simulink model "gm_final_heart_sym2_level4_hdl"  (R2021a)
settings: Solver=FixedStepDiscrete  StartTime=0.0  StopTime=8  RelTol=1e-3
libraries: hdlmdlgenlib x45
(part 2 of 3)

== system gm_final_heart_sym2_level4_hdl/DWT_Sym2_Level4/1st_Level_Decomp/LoD_Even ==
  In_LoD_e : Inport  OutDataTypeStr=fixdt(0, 16, 23)  PortDimensions=1  SampleTime=2.26757369614512e-05
  Add : Sum  AccumDataTypeStr=fixdt(1, 16, 22)  OutDataTypeStr=fixdt(1, 16, 23)  SampleTime=2.26757369614512e-05
  Delay : Delay  DelayLength=double(1)  InitialCondition=0  SampleTime=2.26757369614512e-05
  HwModeRegister{,1..3} (4 alike) : Delay  DelayLength=double(1)  InitialCondition=0  SampleTime=2.26757369614512e-05
  LoD_0 : Constant  Value=-0.1294097900390625  OutDataTypeStr=fixdt(1, 16, 17)  SampleTime=2.26757369614512e-05
  LoD_2 : Constant  Value=0.836517333984375  OutDataTypeStr=fixdt(0, 16, 16)  SampleTime=2.26757369614512e-05
  Multiply : Product  Inputs=**  OutDataTypeStr=fixdt(1, 16, 15)  SampleTime=2.26757369614512e-05
  Multiply1 : Product  Inputs=**  OutDataTypeStr=fixdt(0, 16, 23)  SampleTime=2.26757369614512e-05
  PipelineRegister : Delay  DelayLength=double(1)  InitialCondition=0  SampleTime=2.26757369614512e-05
  PipelineRegister1 : Delay  DelayLength=double(1)  InitialCondition=0  SampleTime=2.26757369614512e-05
  Rate Transition : hdlmdlgenlib/Buffer
      settings: SourceProductBaseCode=SL
  delayMatch : Delay  DelayLength=double(1)  InitialCondition=0  SampleTime=2.26757369614512e-05
  Out_LoD_e : Outport  OutDataTypeStr=fixdt(1,16,23)  SampleTime=2.26757369614512e-05  VectorParamsAs1DForOutWhenUnconnected=off
  wires:
  Add/1 -> Out_LoD_e/1
  Delay/1 -> Rate Transition/1
  LoD_0/1 -> HwModeRegister/1
  LoD_2/1 -> HwModeRegister2/1
  PipelineRegister/1 -> Add/1
  delayMatch/1 -> Add/2
  Rate Transition/1 -> HwModeRegister3/1
  In_LoD_e/1 -> Delay/1, HwModeRegister1/1
  PipelineRegister1/1 -> delayMatch/1
  Multiply/1 -> PipelineRegister/1
  HwModeRegister/1 -> Multiply/1
  HwModeRegister1/1 -> Multiply/2
  Multiply1/1 -> PipelineRegister1/1
  HwModeRegister2/1 -> Multiply1/1
  HwModeRegister3/1 -> Multiply1/2

== system gm_final_heart_sym2_level4_hdl/DWT_Sym2_Level4/1st_Level_Decomp/LoD_Odd ==
  In_LoD_o : Inport  OutDataTypeStr=fixdt(0, 16, 23)  PortDimensions=1  SampleTime=2.26757369614512e-05
  Add : Sum  AccumDataTypeStr=fixdt(0, 16, 24)  OutDataTypeStr=fixdt(0, 16, 24)  SampleTime=2.26757369614512e-05
  Delay : Delay  DelayLength=double(1)  InitialCondition=0  SampleTime=2.26757369614512e-05
  HwModeRegister{,1..3} (4 alike) : Delay  DelayLength=double(1)  InitialCondition=0  SampleTime=2.26757369614512e-05
  LoD_1 : Constant  Value=0.22414398193359375  OutDataTypeStr=fixdt(0, 16, 18)  SampleTime=2.26757369614512e-05
  LoD_3 : Constant  Value=0.48296356201171875  OutDataTypeStr=fixdt(0, 16, 17)  SampleTime=2.26757369614512e-05
  Multiply : Product  Inputs=**  OutDataTypeStr=fixdt(0, 16, 25)  SampleTime=2.26757369614512e-05
  Multiply1 : Product  Inputs=**  OutDataTypeStr=fixdt(0, 16, 24)  SampleTime=2.26757369614512e-05
  PipelineRegister : Delay  DelayLength=double(1)  InitialCondition=0  SampleTime=2.26757369614512e-05
  PipelineRegister1 : Delay  DelayLength=double(1)  InitialCondition=0  SampleTime=2.26757369614512e-05
  Rate Transition : hdlmdlgenlib/Buffer
      settings: SourceProductBaseCode=SL
  delayMatch : Delay  DelayLength=double(1)  InitialCondition=0  SampleTime=2.26757369614512e-05
  Out_LoD_o : Outport  OutDataTypeStr=fixdt(0,16,24)  SampleTime=2.26757369614512e-05  VectorParamsAs1DForOutWhenUnconnected=off
  wires:
  Add/1 -> Out_LoD_o/1
  Delay/1 -> Rate Transition/1
  LoD_1/1 -> HwModeRegister/1
  LoD_3/1 -> HwModeRegister2/1
  PipelineRegister/1 -> Add/1
  delayMatch/1 -> Add/2
  Rate Transition/1 -> HwModeRegister3/1
  In_LoD_o/1 -> Delay/1, HwModeRegister1/1
  PipelineRegister1/1 -> delayMatch/1
  Multiply/1 -> PipelineRegister/1
  HwModeRegister/1 -> Multiply/1
  HwModeRegister1/1 -> Multiply/2
  Multiply1/1 -> PipelineRegister1/1
  HwModeRegister2/1 -> Multiply1/1
  HwModeRegister3/1 -> Multiply1/2

== system gm_final_heart_sym2_level4_hdl/DWT_Sym2_Level4/1st_Level_Decomp1/HiD_Even ==
  In_HiD_e : Inport  OutDataTypeStr=fixdt(1, 16, 22)  PortDimensions=1  SampleTime=2.26757369614512e-05
  Add : Sum  AccumDataTypeStr=fixdt(1, 16, 15)  OutDataTypeStr=fixdt(1, 16, 15)  SampleTime=2.26757369614512e-05
  Delay : Delay  DelayLength=double(1)  InitialCondition=0  SampleTime=2.26757369614512e-05
  HiD_0 : Constant  Value=-0.4829559326171875  OutDataTypeStr=fixdt(1, 16, 16)  SampleTime=2.26757369614512e-05
  HiD_2 : Constant  Value=-0.22414398193359375  OutDataTypeStr=fixdt(1, 16, 17)  SampleTime=2.26757369614512e-05
  HwModeRegister{,1..3} (4 alike) : Delay  DelayLength=double(1)  InitialCondition=0  SampleTime=2.26757369614512e-05
  Multiply : Product  Inputs=**  OutDataTypeStr=fixdt(1, 16, 15)  SampleTime=2.26757369614512e-05
  Multiply1 : Product  Inputs=**  OutDataTypeStr=fixdt(1, 16, 15)  SampleTime=2.26757369614512e-05
  PipelineRegister : Delay  DelayLength=double(1)  InitialCondition=0  SampleTime=2.26757369614512e-05
  PipelineRegister1 : Delay  DelayLength=double(1)  InitialCondition=0  SampleTime=2.26757369614512e-05
  Rate Transition : hdlmdlgenlib/Buffer
      settings: SourceProductBaseCode=SL
  delayMatch : Delay  DelayLength=double(1)  InitialCondition=0  SampleTime=2.26757369614512e-05
  Out_HiD_e : Outport  OutDataTypeStr=fixdt(1,16,15)  SampleTime=2.26757369614512e-05  VectorParamsAs1DForOutWhenUnconnected=off
  wires:
  Add/1 -> Out_HiD_e/1
  Delay/1 -> Rate Transition/1
  HiD_0/1 -> HwModeRegister/1
  HiD_2/1 -> HwModeRegister2/1
  PipelineRegister/1 -> Add/1
  delayMatch/1 -> Add/2
  Rate Transition/1 -> HwModeRegister3/1
  In_HiD_e/1 -> Delay/1, HwModeRegister1/1
  PipelineRegister1/1 -> delayMatch/1
  Multiply/1 -> PipelineRegister/1
  HwModeRegister/1 -> Multiply/1
  HwModeRegister1/1 -> Multiply/2
  Multiply1/1 -> PipelineRegister1/1
  HwModeRegister2/1 -> Multiply1/1
  HwModeRegister3/1 -> Multiply1/2

== system gm_final_heart_sym2_level4_hdl/DWT_Sym2_Level4/1st_Level_Decomp1/HiD_Odd ==
  In_HiD_o : Inport  OutDataTypeStr=fixdt(1, 16, 22)  PortDimensions=1  SampleTime=2.26757369614512e-05
  Add : Sum  AccumDataTypeStr=fixdt(1, 16, 23)  OutDataTypeStr=fixdt(1, 16, 23)  SampleTime=2.26757369614512e-05
  Delay : Delay  DelayLength=double(1)  InitialCondition=0  SampleTime=2.26757369614512e-05
  HiD_1 : Constant  Value=0.836517333984375  OutDataTypeStr=fixdt(0, 16, 16)  SampleTime=2.26757369614512e-05
  HiD_3 : Constant  Value=-0.1294097900390625  OutDataTypeStr=fixdt(1, 16, 17)  SampleTime=2.26757369614512e-05
  HwModeRegister{,1..3} (4 alike) : Delay  DelayLength=double(1)  InitialCondition=0  SampleTime=2.26757369614512e-05
  Multiply : Product  Inputs=**  OutDataTypeStr=fixdt(0, 16, 24)  SampleTime=2.26757369614512e-05
  Multiply1 : Product  Inputs=**  OutDataTypeStr=fixdt(1, 16, 15)  SampleTime=2.26757369614512e-05
  PipelineRegister : Delay  DelayLength=double(1)  InitialCondition=0  SampleTime=2.26757369614512e-05
  PipelineRegister1 : Delay  DelayLength=double(1)  InitialCondition=0  SampleTime=2.26757369614512e-05
  Rate Transition : hdlmdlgenlib/Buffer
      settings: SourceProductBaseCode=SL
  delayMatch : Delay  DelayLength=double(1)  InitialCondition=0  SampleTime=2.26757369614512e-05
  Out_HiD_o : Outport  OutDataTypeStr=fixdt(1,16,23)  SampleTime=2.26757369614512e-05  VectorParamsAs1DForOutWhenUnconnected=off
  wires:
  Add/1 -> Out_HiD_o/1
  Delay/1 -> Rate Transition/1
  HiD_1/1 -> HwModeRegister/1
  HiD_3/1 -> HwModeRegister2/1
  PipelineRegister/1 -> Add/1
  delayMatch/1 -> Add/2
  Rate Transition/1 -> HwModeRegister3/1
  In_HiD_o/1 -> Delay/1, HwModeRegister1/1
  PipelineRegister1/1 -> delayMatch/1
  Multiply/1 -> PipelineRegister/1
  HwModeRegister/1 -> Multiply/1
  HwModeRegister1/1 -> Multiply/2
  Multiply1/1 -> PipelineRegister1/1
  HwModeRegister2/1 -> Multiply1/1
  HwModeRegister3/1 -> Multiply1/2

== system gm_final_heart_sym2_level4_hdl/DWT_Sym2_Level4/1st_Level_Decomp1/LoD_Even ==
  In_LoD_e : Inport  OutDataTypeStr=fixdt(1, 16, 22)  PortDimensions=1  SampleTime=2.26757369614512e-05
  Add : Sum  AccumDataTypeStr=fixdt(1, 16, 23)  OutDataTypeStr=fixdt(1, 16, 23)  SampleTime=2.26757369614512e-05
  Delay : Delay  DelayLength=double(1)  InitialCondition=0  SampleTime=2.26757369614512e-05
  HwModeRegister{,1..3} (4 alike) : Delay  DelayLength=double(1)  InitialCondition=0  SampleTime=2.26757369614512e-05
  LoD_0 : Constant  Value=-0.1294097900390625  OutDataTypeStr=fixdt(1, 16, 17)  SampleTime=2.26757369614512e-05
  LoD_2 : Constant  Value=0.836517333984375  OutDataTypeStr=fixdt(0, 16, 16)  SampleTime=2.26757369614512e-05
  Multiply : Product  Inputs=**  OutDataTypeStr=fixdt(1, 16, 15)  SampleTime=2.26757369614512e-05
  Multiply1 : Product  Inputs=**  OutDataTypeStr=fixdt(0, 16, 24)  SampleTime=2.26757369614512e-05
  PipelineRegister : Delay  DelayLength=double(1)  InitialCondition=0  SampleTime=2.26757369614512e-05
  PipelineRegister1 : Delay  DelayLength=double(1)  InitialCondition=0  SampleTime=2.26757369614512e-05
  Rate Transition : hdlmdlgenlib/Buffer
      settings: SourceProductBaseCode=SL
  delayMatch : Delay  DelayLength=double(1)  InitialCondition=0  SampleTime=2.26757369614512e-05
  Out_LoD_e : Outport  OutDataTypeStr=fixdt(1,16,23)  SampleTime=2.26757369614512e-05  VectorParamsAs1DForOutWhenUnconnected=off
  wires:
  Add/1 -> Out_LoD_e/1
  Delay/1 -> Rate Transition/1
  LoD_0/1 -> HwModeRegister/1
  LoD_2/1 -> HwModeRegister2/1
  PipelineRegister/1 -> Add/1
  delayMatch/1 -> Add/2
  Rate Transition/1 -> HwModeRegister3/1
  In_LoD_e/1 -> Delay/1, HwModeRegister1/1
  PipelineRegister1/1 -> delayMatch/1
  Multiply/1 -> PipelineRegister/1
  HwModeRegister/1 -> Multiply/1
  HwModeRegister1/1 -> Multiply/2
  Multiply1/1 -> PipelineRegister1/1
  HwModeRegister2/1 -> Multiply1/1
  HwModeRegister3/1 -> Multiply1/2

== system gm_final_heart_sym2_level4_hdl/DWT_Sym2_Level4/1st_Level_Decomp1/LoD_Odd ==
  In_LoD_o : Inport  OutDataTypeStr=fixdt(1, 16, 22)  PortDimensions=1  SampleTime=2.26757369614512e-05
  Add : Sum  AccumDataTypeStr=fixdt(0, 16, 24)  OutDataTypeStr=fixdt(0, 16, 24)  SampleTime=2.26757369614512e-05
  Delay : Delay  DelayLength=double(1)  InitialCondition=0  SampleTime=2.26757369614512e-05
  HwModeRegister{,1..3} (4 alike) : Delay  DelayLength=double(1)  InitialCondition=0  SampleTime=2.26757369614512e-05
  LoD_1 : Constant  Value=0.22414398193359375  OutDataTypeStr=fixdt(0, 16, 18)  SampleTime=2.26757369614512e-05
  LoD_3 : Constant  Value=0.48296356201171875  OutDataTypeStr=fixdt(0, 16, 17)  SampleTime=2.26757369614512e-05
  Multiply : Product  Inputs=**  OutDataTypeStr=fixdt(0, 16, 26)  SampleTime=2.26757369614512e-05
  Multiply1 : Product  Inputs=**  OutDataTypeStr=fixdt(0, 16, 25)  SampleTime=2.26757369614512e-05
  PipelineRegister : Delay  DelayLength=double(1)  InitialCondition=0  SampleTime=2.26757369614512e-05
  PipelineRegister1 : Delay  DelayLength=double(1)  InitialCondition=0  SampleTime=2.26757369614512e-05
  Rate Transition : hdlmdlgenlib/Buffer
      settings: SourceProductBaseCode=SL
  delayMatch : Delay  DelayLength=double(1)  InitialCondition=0  SampleTime=2.26757369614512e-05
  Out_LoD_o : Outport  OutDataTypeStr=fixdt(0,16,24)  SampleTime=2.26757369614512e-05  VectorParamsAs1DForOutWhenUnconnected=off
  wires:
  Add/1 -> Out_LoD_o/1
  Delay/1 -> Rate Transition/1
  LoD_1/1 -> HwModeRegister/1
  LoD_3/1 -> HwModeRegister2/1
  PipelineRegister/1 -> Add/1
  delayMatch/1 -> Add/2
  Rate Transition/1 -> HwModeRegister3/1
  In_LoD_o/1 -> Delay/1, HwModeRegister1/1
  PipelineRegister1/1 -> delayMatch/1
  Multiply/1 -> PipelineRegister/1
  HwModeRegister/1 -> Multiply/1
  HwModeRegister1/1 -> Multiply/2
  Multiply1/1 -> PipelineRegister1/1
  HwModeRegister2/1 -> Multiply1/1
  HwModeRegister3/1 -> Multiply1/2

== system gm_final_heart_sym2_level4_hdl/DWT_Sym2_Level4/1st_Level_Decomp2/HiD_Even ==
  In_HiD_e : Inport  OutDataTypeStr=fixdt(0, 16, 24)  PortDimensions=1  SampleTime=2.26757369614512e-05
  Add : Sum  AccumDataTypeStr=fixdt(1, 16, 15)  OutDataTypeStr=fixdt(1, 16, 15)  SampleTime=2.26757369614512e-05
  Delay : Delay  DelayLength=double(1)  InitialCondition=0  SampleTime=2.26757369614512e-05
  HiD_0 : Constant  Value=-0.4829559326171875  OutDataTypeStr=fixdt(1, 16, 16)  SampleTime=2.26757369614512e-05
  HiD_2 : Constant  Value=-0.22414398193359375  OutDataTypeStr=fixdt(1, 16, 17)  SampleTime=2.26757369614512e-05
  HwModeRegister{,1..3} (4 alike) : Delay  DelayLength=double(1)  InitialCondition=0  SampleTime=2.26757369614512e-05
  Multiply : Product  Inputs=**  OutDataTypeStr=fixdt(1, 16, 15)  SampleTime=2.26757369614512e-05
  Multiply1 : Product  Inputs=**  OutDataTypeStr=fixdt(1, 16, 15)  SampleTime=2.26757369614512e-05
  PipelineRegister : Delay  DelayLength=double(1)  InitialCondition=0  SampleTime=2.26757369614512e-05
  PipelineRegister1 : Delay  DelayLength=double(1)  InitialCondition=0  SampleTime=2.26757369614512e-05
  Rate Transition : hdlmdlgenlib/Buffer
      settings: SourceProductBaseCode=SL
  delayMatch : Delay  DelayLength=double(1)  InitialCondition=0  SampleTime=2.26757369614512e-05
  Out_HiD_e : Outport  OutDataTypeStr=fixdt(1,16,15)  SampleTime=2.26757369614512e-05  VectorParamsAs1DForOutWhenUnconnected=off
  wires:
  Add/1 -> Out_HiD_e/1
  Delay/1 -> Rate Transition/1
  HiD_0/1 -> HwModeRegister/1
  HiD_2/1 -> HwModeRegister2/1
  PipelineRegister/1 -> Add/1
  delayMatch/1 -> Add/2
  Rate Transition/1 -> HwModeRegister3/1
  In_HiD_e/1 -> Delay/1, HwModeRegister1/1
  PipelineRegister1/1 -> delayMatch/1
  Multiply/1 -> PipelineRegister/1
  HwModeRegister/1 -> Multiply/1
  HwModeRegister1/1 -> Multiply/2
  Multiply1/1 -> PipelineRegister1/1
  HwModeRegister2/1 -> Multiply1/1
  HwModeRegister3/1 -> Multiply1/2

== system gm_final_heart_sym2_level4_hdl/DWT_Sym2_Level4/1st_Level_Decomp2/HiD_Odd ==
  In_HiD_o : Inport  OutDataTypeStr=fixdt(0, 16, 24)  PortDimensions=1  SampleTime=2.26757369614512e-05
  Add : Sum  AccumDataTypeStr=fixdt(1, 16, 23)  OutDataTypeStr=fixdt(1, 16, 23)  SampleTime=2.26757369614512e-05
  Delay : Delay  DelayLength=double(1)  InitialCondition=0  SampleTime=2.26757369614512e-05
  HiD_1 : Constant  Value=0.836517333984375  OutDataTypeStr=fixdt(0, 16, 16)  SampleTime=2.26757369614512e-05
  HiD_3 : Constant  Value=-0.1294097900390625  OutDataTypeStr=fixdt(1, 16, 17)  SampleTime=2.26757369614512e-05
  HwModeRegister{,1..3} (4 alike) : Delay  DelayLength=double(1)  InitialCondition=0  SampleTime=2.26757369614512e-05
  Multiply : Product  Inputs=**  OutDataTypeStr=fixdt(0, 16, 24)  SampleTime=2.26757369614512e-05
  Multiply1 : Product  Inputs=**  OutDataTypeStr=fixdt(1, 16, 15)  SampleTime=2.26757369614512e-05
  PipelineRegister : Delay  DelayLength=double(1)  InitialCondition=0  SampleTime=2.26757369614512e-05
  PipelineRegister1 : Delay  DelayLength=double(1)  InitialCondition=0  SampleTime=2.26757369614512e-05
  Rate Transition : hdlmdlgenlib/Buffer
      settings: SourceProductBaseCode=SL
  delayMatch : Delay  DelayLength=double(1)  InitialCondition=0  SampleTime=2.26757369614512e-05
  Out_HiD_o : Outport  OutDataTypeStr=fixdt(1,16,23)  SampleTime=2.26757369614512e-05  VectorParamsAs1DForOutWhenUnconnected=off
  wires:
  Add/1 -> Out_HiD_o/1
  Delay/1 -> Rate Transition/1
  HiD_1/1 -> HwModeRegister/1
  HiD_3/1 -> HwModeRegister2/1
  PipelineRegister/1 -> Add/1
  delayMatch/1 -> Add/2
  Rate Transition/1 -> HwModeRegister3/1
  In_HiD_o/1 -> Delay/1, HwModeRegister1/1
  PipelineRegister1/1 -> delayMatch/1
  Multiply/1 -> PipelineRegister/1
  HwModeRegister/1 -> Multiply/1
  HwModeRegister1/1 -> Multiply/2
  Multiply1/1 -> PipelineRegister1/1
  HwModeRegister2/1 -> Multiply1/1
  HwModeRegister3/1 -> Multiply1/2

== system gm_final_heart_sym2_level4_hdl/DWT_Sym2_Level4/1st_Level_Decomp2/LoD_Even ==
  In_LoD_e : Inport  OutDataTypeStr=fixdt(0, 16, 24)  PortDimensions=1  SampleTime=2.26757369614512e-05
  Add : Sum  AccumDataTypeStr=fixdt(1, 16, 23)  OutDataTypeStr=fixdt(1, 16, 23)  SampleTime=2.26757369614512e-05
  Delay : Delay  DelayLength=double(1)  InitialCondition=0  SampleTime=2.26757369614512e-05
  HwModeRegister{,1..3} (4 alike) : Delay  DelayLength=double(1)  InitialCondition=0  SampleTime=2.26757369614512e-05
  LoD_0 : Constant  Value=-0.1294097900390625  OutDataTypeStr=fixdt(1, 16, 17)  SampleTime=2.26757369614512e-05
  LoD_2 : Constant  Value=0.836517333984375  OutDataTypeStr=fixdt(0, 16, 16)  SampleTime=2.26757369614512e-05
  Multiply : Product  Inputs=**  OutDataTypeStr=fixdt(1, 16, 15)  SampleTime=2.26757369614512e-05
  Multiply1 : Product  Inputs=**  OutDataTypeStr=fixdt(0, 16, 24)  SampleTime=2.26757369614512e-05
  PipelineRegister : Delay  DelayLength=double(1)  InitialCondition=0  SampleTime=2.26757369614512e-05
  PipelineRegister1 : Delay  DelayLength=double(1)  InitialCondition=0  SampleTime=2.26757369614512e-05
  Rate Transition : hdlmdlgenlib/Buffer
      settings: SourceProductBaseCode=SL
  delayMatch : Delay  DelayLength=double(1)  InitialCondition=0  SampleTime=2.26757369614512e-05
  Out_LoD_e : Outport  OutDataTypeStr=fixdt(1,16,23)  SampleTime=2.26757369614512e-05  VectorParamsAs1DForOutWhenUnconnected=off
  wires:
  Add/1 -> Out_LoD_e/1
  Delay/1 -> Rate Transition/1
  LoD_0/1 -> HwModeRegister/1
  LoD_2/1 -> HwModeRegister2/1
  PipelineRegister/1 -> Add/1
  delayMatch/1 -> Add/2
  Rate Transition/1 -> HwModeRegister3/1
  In_LoD_e/1 -> Delay/1, HwModeRegister1/1
  PipelineRegister1/1 -> delayMatch/1
  Multiply/1 -> PipelineRegister/1
  HwModeRegister/1 -> Multiply/1
  HwModeRegister1/1 -> Multiply/2
  Multiply1/1 -> PipelineRegister1/1
  HwModeRegister2/1 -> Multiply1/1
  HwModeRegister3/1 -> Multiply1/2

== system gm_final_heart_sym2_level4_hdl/DWT_Sym2_Level4/1st_Level_Decomp2/LoD_Odd ==
  In_LoD_o : Inport  OutDataTypeStr=fixdt(0, 16, 24)  PortDimensions=1  SampleTime=2.26757369614512e-05
  Add : Sum  AccumDataTypeStr=fixdt(0, 16, 24)  OutDataTypeStr=fixdt(0, 16, 24)  SampleTime=2.26757369614512e-05
  Delay : Delay  DelayLength=double(1)  InitialCondition=0  SampleTime=2.26757369614512e-05
  HwModeRegister{,1..3} (4 alike) : Delay  DelayLength=double(1)  InitialCondition=0  SampleTime=2.26757369614512e-05
  LoD_1 : Constant  Value=0.22414398193359375  OutDataTypeStr=fixdt(0, 16, 18)  SampleTime=2.26757369614512e-05
  LoD_3 : Constant  Value=0.48296356201171875  OutDataTypeStr=fixdt(0, 16, 17)  SampleTime=2.26757369614512e-05
  Multiply : Product  Inputs=**  OutDataTypeStr=fixdt(0, 16, 26)  SampleTime=2.26757369614512e-05
  Multiply1 : Product  Inputs=**  OutDataTypeStr=fixdt(0, 16, 25)  SampleTime=2.26757369614512e-05
  PipelineRegister : Delay  DelayLength=double(1)  InitialCondition=0  SampleTime=2.26757369614512e-05
  PipelineRegister1 : Delay  DelayLength=double(1)  InitialCondition=0  SampleTime=2.26757369614512e-05
  Rate Transition : hdlmdlgenlib/Buffer
      settings: SourceProductBaseCode=SL
  delayMatch : Delay  DelayLength=double(1)  InitialCondition=0  SampleTime=2.26757369614512e-05
  Out_LoD_o : Outport  OutDataTypeStr=fixdt(0,16,24)  SampleTime=2.26757369614512e-05  VectorParamsAs1DForOutWhenUnconnected=off
  wires:
  Add/1 -> Out_LoD_o/1
  Delay/1 -> Rate Transition/1
  LoD_1/1 -> HwModeRegister/1
  LoD_3/1 -> HwModeRegister2/1
  PipelineRegister/1 -> Add/1
  delayMatch/1 -> Add/2
  Rate Transition/1 -> HwModeRegister3/1
  In_LoD_o/1 -> Delay/1, HwModeRegister1/1
  PipelineRegister1/1 -> delayMatch/1
  Multiply/1 -> PipelineRegister/1
  HwModeRegister/1 -> Multiply/1
  HwModeRegister1/1 -> Multiply/2
  Multiply1/1 -> PipelineRegister1/1
  HwModeRegister2/1 -> Multiply1/1
  HwModeRegister3/1 -> Multiply1/2

== system gm_final_heart_sym2_level4_hdl/DWT_Sym2_Level4/1st_Level_Decomp3/HiD_Even ==
  In_HiD_e : Inport  OutDataTypeStr=fixdt(0, 16, 24)  PortDimensions=1  SampleTime=2.26757369614512e-05
  Add : Sum  AccumDataTypeStr=fixdt(1, 16, 15)  OutDataTypeStr=fixdt(1, 16, 15)  SampleTime=2.26757369614512e-05
  Delay : Delay  DelayLength=double(1)  InitialCondition=0  SampleTime=2.26757369614512e-05
  HiD_0 : Constant  Value=-0.4829559326171875  OutDataTypeStr=fixdt(1, 16, 16)  SampleTime=2.26757369614512e-05
  HiD_2 : Constant  Value=-0.22414398193359375  OutDataTypeStr=fixdt(1, 16, 17)  SampleTime=2.26757369614512e-05
  HwModeRegister{,1..3} (4 alike) : Delay  DelayLength=double(1)  InitialCondition=0  SampleTime=2.26757369614512e-05
  Multiply : Product  Inputs=**  OutDataTypeStr=fixdt(1, 16, 15)  SampleTime=2.26757369614512e-05
  Multiply1 : Product  Inputs=**  OutDataTypeStr=fixdt(1, 16, 15)  SampleTime=2.26757369614512e-05
  PipelineRegister : Delay  DelayLength=double(1)  InitialCondition=0  SampleTime=2.26757369614512e-05
  PipelineRegister1 : Delay  DelayLength=double(1)  InitialCondition=0  SampleTime=2.26757369614512e-05
  Rate Transition : hdlmdlgenlib/Buffer
      settings: SourceProductBaseCode=SL
  delayMatch : Delay  DelayLength=double(1)  InitialCondition=0  SampleTime=2.26757369614512e-05
  Out_HiD_e : Outport  OutDataTypeStr=fixdt(1,16,15)  SampleTime=2.26757369614512e-05  VectorParamsAs1DForOutWhenUnconnected=off
  wires:
  Add/1 -> Out_HiD_e/1
  Delay/1 -> Rate Transition/1
  HiD_0/1 -> HwModeRegister/1
  HiD_2/1 -> HwModeRegister2/1
  PipelineRegister/1 -> Add/1
  delayMatch/1 -> Add/2
  Rate Transition/1 -> HwModeRegister3/1
  In_HiD_e/1 -> Delay/1, HwModeRegister1/1
  PipelineRegister1/1 -> delayMatch/1
  Multiply/1 -> PipelineRegister/1
  HwModeRegister/1 -> Multiply/1
  HwModeRegister1/1 -> Multiply/2
  Multiply1/1 -> PipelineRegister1/1
  HwModeRegister2/1 -> Multiply1/1
  HwModeRegister3/1 -> Multiply1/2

== system gm_final_heart_sym2_level4_hdl/DWT_Sym2_Level4/1st_Level_Decomp3/HiD_Odd ==
  In_HiD_o : Inport  OutDataTypeStr=fixdt(0, 16, 24)  PortDimensions=1  SampleTime=2.26757369614512e-05
  Add : Sum  AccumDataTypeStr=fixdt(1, 16, 23)  OutDataTypeStr=fixdt(1, 16, 23)  SampleTime=2.26757369614512e-05
  Delay : Delay  DelayLength=double(1)  InitialCondition=0  SampleTime=2.26757369614512e-05
  HiD_1 : Constant  Value=0.836517333984375  OutDataTypeStr=fixdt(0, 16, 16)  SampleTime=2.26757369614512e-05
  HiD_3 : Constant  Value=-0.1294097900390625  OutDataTypeStr=fixdt(1, 16, 17)  SampleTime=2.26757369614512e-05
  HwModeRegister{,1..3} (4 alike) : Delay  DelayLength=double(1)  InitialCondition=0  SampleTime=2.26757369614512e-05
  Multiply : Product  Inputs=**  OutDataTypeStr=fixdt(0, 16, 24)  SampleTime=2.26757369614512e-05
  Multiply1 : Product  Inputs=**  OutDataTypeStr=fixdt(1, 16, 15)  SampleTime=2.26757369614512e-05
  PipelineRegister : Delay  DelayLength=double(1)  InitialCondition=0  SampleTime=2.26757369614512e-05
  PipelineRegister1 : Delay  DelayLength=double(1)  InitialCondition=0  SampleTime=2.26757369614512e-05
  Rate Transition : hdlmdlgenlib/Buffer
      settings: SourceProductBaseCode=SL
  delayMatch : Delay  DelayLength=double(1)  InitialCondition=0  SampleTime=2.26757369614512e-05
  Out_HiD_o : Outport  OutDataTypeStr=fixdt(1,16,23)  SampleTime=2.26757369614512e-05  VectorParamsAs1DForOutWhenUnconnected=off
  wires:
  Add/1 -> Out_HiD_o/1
  Delay/1 -> Rate Transition/1
  HiD_1/1 -> HwModeRegister/1
  HiD_3/1 -> HwModeRegister2/1
  PipelineRegister/1 -> Add/1
  delayMatch/1 -> Add/2
  Rate Transition/1 -> HwModeRegister3/1
  In_HiD_o/1 -> Delay/1, HwModeRegister1/1
  PipelineRegister1/1 -> delayMatch/1
  Multiply/1 -> PipelineRegister/1
  HwModeRegister/1 -> Multiply/1
  HwModeRegister1/1 -> Multiply/2
  Multiply1/1 -> PipelineRegister1/1
  HwModeRegister2/1 -> Multiply1/1
  HwModeRegister3/1 -> Multiply1/2

== system gm_final_heart_sym2_level4_hdl/DWT_Sym2_Level4/1st_Level_Decomp3/LoD_Even ==
  In_LoD_e : Inport  OutDataTypeStr=fixdt(0, 16, 24)  PortDimensions=1  SampleTime=2.26757369614512e-05
  Add : Sum  AccumDataTypeStr=fixdt(1, 16, 23)  OutDataTypeStr=fixdt(1, 16, 23)  SampleTime=2.26757369614512e-05
  Delay : Delay  DelayLength=double(1)  InitialCondition=0  SampleTime=2.26757369614512e-05
  HwModeRegister{,1..3} (4 alike) : Delay  DelayLength=double(1)  InitialCondition=0  SampleTime=2.26757369614512e-05
  LoD_0 : Constant  Value=-0.1294097900390625  OutDataTypeStr=fixdt(1, 16, 17)  SampleTime=2.26757369614512e-05
  LoD_2 : Constant  Value=0.836517333984375  OutDataTypeStr=fixdt(0, 16, 16)  SampleTime=2.26757369614512e-05
  Multiply : Product  Inputs=**  OutDataTypeStr=fixdt(1, 16, 15)  SampleTime=2.26757369614512e-05
  Multiply1 : Product  Inputs=**  OutDataTypeStr=fixdt(0, 16, 24)  SampleTime=2.26757369614512e-05
  PipelineRegister : Delay  DelayLength=double(1)  InitialCondition=0  SampleTime=2.26757369614512e-05
  PipelineRegister1 : Delay  DelayLength=double(1)  InitialCondition=0  SampleTime=2.26757369614512e-05
  Rate Transition : hdlmdlgenlib/Buffer
      settings: SourceProductBaseCode=SL
  delayMatch : Delay  DelayLength=double(1)  InitialCondition=0  SampleTime=2.26757369614512e-05
  Out_LoD_e : Outport  OutDataTypeStr=fixdt(1,16,23)  SampleTime=2.26757369614512e-05  VectorParamsAs1DForOutWhenUnconnected=off
  wires:
  Add/1 -> Out_LoD_e/1
  Delay/1 -> Rate Transition/1
  LoD_0/1 -> HwModeRegister/1
  LoD_2/1 -> HwModeRegister2/1
  PipelineRegister/1 -> Add/1
  delayMatch/1 -> Add/2
  Rate Transition/1 -> HwModeRegister3/1
  In_LoD_e/1 -> Delay/1, HwModeRegister1/1
  PipelineRegister1/1 -> delayMatch/1
  Multiply/1 -> PipelineRegister/1
  HwModeRegister/1 -> Multiply/1
  HwModeRegister1/1 -> Multiply/2
  Multiply1/1 -> PipelineRegister1/1
  HwModeRegister2/1 -> Multiply1/1
  HwModeRegister3/1 -> Multiply1/2

== system gm_final_heart_sym2_level4_hdl/DWT_Sym2_Level4/1st_Level_Decomp3/LoD_Odd ==
  In_LoD_o : Inport  OutDataTypeStr=fixdt(0, 16, 24)  PortDimensions=1  SampleTime=2.26757369614512e-05
  Add : Sum  AccumDataTypeStr=fixdt(0, 16, 24)  OutDataTypeStr=fixdt(0, 16, 24)  SampleTime=2.26757369614512e-05
  Delay : Delay  DelayLength=double(1)  InitialCondition=0  SampleTime=2.26757369614512e-05
  HwModeRegister{,1..3} (4 alike) : Delay  DelayLength=double(1)  InitialCondition=0  SampleTime=2.26757369614512e-05
  LoD_1 : Constant  Value=0.22414398193359375  OutDataTypeStr=fixdt(0, 16, 18)  SampleTime=2.26757369614512e-05
  LoD_3 : Constant  Value=0.48296356201171875  OutDataTypeStr=fixdt(0, 16, 17)  SampleTime=2.26757369614512e-05
  Multiply : Product  Inputs=**  OutDataTypeStr=fixdt(0, 16, 26)  SampleTime=2.26757369614512e-05
  Multiply1 : Product  Inputs=**  OutDataTypeStr=fixdt(0, 16, 25)  SampleTime=2.26757369614512e-05
  PipelineRegister : Delay  DelayLength=double(1)  InitialCondition=0  SampleTime=2.26757369614512e-05
  PipelineRegister1 : Delay  DelayLength=double(1)  InitialCondition=0  SampleTime=2.26757369614512e-05
  Rate Transition : hdlmdlgenlib/Buffer
      settings: SourceProductBaseCode=SL
  delayMatch : Delay  DelayLength=double(1)  InitialCondition=0  SampleTime=2.26757369614512e-05
  Out_LoD_o : Outport  OutDataTypeStr=fixdt(0,16,24)  SampleTime=2.26757369614512e-05  VectorParamsAs1DForOutWhenUnconnected=off
  wires:
  Add/1 -> Out_LoD_o/1
  Delay/1 -> Rate Transition/1
  LoD_1/1 -> HwModeRegister/1
  LoD_3/1 -> HwModeRegister2/1
  PipelineRegister/1 -> Add/1
  delayMatch/1 -> Add/2
  Rate Transition/1 -> HwModeRegister3/1
  In_LoD_o/1 -> Delay/1, HwModeRegister1/1
  PipelineRegister1/1 -> delayMatch/1
  Multiply/1 -> PipelineRegister/1
  HwModeRegister/1 -> Multiply/1
  HwModeRegister1/1 -> Multiply/2
  Multiply1/1 -> PipelineRegister1/1
  HwModeRegister2/1 -> Multiply1/1
  HwModeRegister3/1 -> Multiply1/2

== system gm_final_heart_sym2_level4_hdl/DWT_Sym2_Level4/1st_Level_Recon/HiR_Even ==
  In_HiR_e : Inport  OutDataTypeStr=fixdt(1, 16, 27)  PortDimensions=1  SampleTime=2.26757369614512e-05
  Add : Sum  AccumDataTypeStr=fixdt(1, 16, 28)  OutDataTypeStr=fixdt(1, 16, 28)  SampleTime=2.26757369614512e-05
  Constant12 : Constant  Value=-0.1294097900390625  OutDataTypeStr=fixdt(1, 16, 17)  SampleTime=2.26757369614512e-05
  Constant14 : Constant  Value=0.836517333984375  OutDataTypeStr=fixdt(0, 16, 16)  SampleTime=2.26757369614512e-05
  Delay : Delay  DelayLength=double(1)  InitialCondition=0  SampleTime=2.26757369614512e-05
  HwModeRegister{,1..3} (4 alike) : Delay  DelayLength=double(1)  InitialCondition=0  SampleTime=2.26757369614512e-05
  Multiply : Product  Inputs=**  OutDataTypeStr=fixdt(1, 16, 30)  SampleTime=2.26757369614512e-05
  Multiply1 : Product  Inputs=**  OutDataTypeStr=fixdt(1, 16, 28)  SampleTime=2.26757369614512e-05
  PipelineRegister : Delay  DelayLength=double(1)  InitialCondition=0  SampleTime=2.26757369614512e-05
  PipelineRegister1 : Delay  DelayLength=double(1)  InitialCondition=0  SampleTime=2.26757369614512e-05
  Rate Transition : hdlmdlgenlib/Buffer
      settings: SourceProductBaseCode=SL
  delayMatch : Delay  DelayLength=double(1)  InitialCondition=0  SampleTime=2.26757369614512e-05
  Out_HiR_e : Outport  OutDataTypeStr=fixdt(1,16,28)  SampleTime=2.26757369614512e-05  VectorParamsAs1DForOutWhenUnconnected=off
  wires:
  Add/1 -> Out_HiR_e/1
  Constant12/1 -> HwModeRegister/1
  Constant14/1 -> HwModeRegister2/1
  Delay/1 -> Rate Transition/1
  PipelineRegister/1 -> Add/1
  delayMatch/1 -> Add/2
  Rate Transition/1 -> HwModeRegister3/1
  In_HiR_e/1 -> Delay/1, HwModeRegister1/1
  PipelineRegister1/1 -> delayMatch/1
  Multiply/1 -> PipelineRegister/1
  HwModeRegister/1 -> Multiply/1
  HwModeRegister1/1 -> Multiply/2
  Multiply1/1 -> PipelineRegister1/1
  HwModeRegister2/1 -> Multiply1/1
  HwModeRegister3/1 -> Multiply1/2

== system gm_final_heart_sym2_level4_hdl/DWT_Sym2_Level4/1st_Level_Recon/HiR_Odd ==
  In_HiR_o : Inport  OutDataTypeStr=fixdt(1, 16, 27)  PortDimensions=1  SampleTime=2.26757369614512e-05
  Add : Sum  AccumDataTypeStr=fixdt(1, 16, 29)  OutDataTypeStr=fixdt(1, 16, 29)  SampleTime=2.26757369614512e-05
  Constant13 : Constant  Value=-0.22414398193359375  OutDataTypeStr=fixdt(1, 16, 17)  SampleTime=2.26757369614512e-05
  Constant15 : Constant  Value=-0.4829559326171875  OutDataTypeStr=fixdt(1, 16, 16)  SampleTime=2.26757369614512e-05
  Delay : Delay  DelayLength=double(1)  InitialCondition=0  SampleTime=2.26757369614512e-05
  HwModeRegister{,1..3} (4 alike) : Delay  DelayLength=double(1)  InitialCondition=0  SampleTime=2.26757369614512e-05
  Multiply : Product  Inputs=**  OutDataTypeStr=fixdt(1, 16, 30)  SampleTime=2.26757369614512e-05
  Multiply1 : Product  Inputs=**  OutDataTypeStr=fixdt(1, 16, 29)  SampleTime=2.26757369614512e-05
  PipelineRegister : Delay  DelayLength=double(1)  InitialCondition=0  SampleTime=2.26757369614512e-05
  PipelineRegister1 : Delay  DelayLength=double(1)  InitialCondition=0  SampleTime=2.26757369614512e-05
  Rate Transition : hdlmdlgenlib/Buffer
      settings: SourceProductBaseCode=SL
  delayMatch : Delay  DelayLength=double(1)  InitialCondition=0  SampleTime=2.26757369614512e-05
  Out_HiR_o : Outport  OutDataTypeStr=fixdt(1,16,29)  SampleTime=2.26757369614512e-05  VectorParamsAs1DForOutWhenUnconnected=off
  wires:
  Add/1 -> Out_HiR_o/1
  Constant13/1 -> HwModeRegister/1
  Constant15/1 -> HwModeRegister2/1
  Delay/1 -> Rate Transition/1
  PipelineRegister/1 -> Add/1
  delayMatch/1 -> Add/2
  Rate Transition/1 -> HwModeRegister3/1
  In_HiR_o/1 -> Delay/1, HwModeRegister1/1
  PipelineRegister1/1 -> delayMatch/1
  Multiply/1 -> PipelineRegister/1
  HwModeRegister/1 -> Multiply/1
  HwModeRegister1/1 -> Multiply/2
  Multiply1/1 -> PipelineRegister1/1
  HwModeRegister2/1 -> Multiply1/1
  HwModeRegister3/1 -> Multiply1/2

== system gm_final_heart_sym2_level4_hdl/DWT_Sym2_Level4/1st_Level_Recon/LoR_Even ==
  In_LoR_e : Inport  OutDataTypeStr=fixdt(0, 16, 24)  PortDimensions=1  SampleTime=2.26757369614512e-05
  Add : Sum  AccumDataTypeStr=fixdt(0, 16, 25)  OutDataTypeStr=fixdt(0, 16, 25)  SampleTime=2.26757369614512e-05
  Constant10 : Constant  Value=0.22414398193359375  OutDataTypeStr=fixdt(0, 16, 18)  SampleTime=2.26757369614512e-05
  Constant8 : Constant  Value=0.48296356201171875  OutDataTypeStr=fixdt(0, 16, 17)  SampleTime=2.26757369614512e-05
  Delay : Delay  DelayLength=double(1)  InitialCondition=0  SampleTime=2.26757369614512e-05
  HwModeRegister{,1..3} (4 alike) : Delay  DelayLength=double(1)  InitialCondition=0  SampleTime=2.26757369614512e-05
  Multiply : Product  Inputs=**  OutDataTypeStr=fixdt(0, 16, 25)  SampleTime=2.26757369614512e-05
  Multiply1 : Product  Inputs=**  OutDataTypeStr=fixdt(0, 16, 26)  SampleTime=2.26757369614512e-05
  PipelineRegister : Delay  DelayLength=double(1)  InitialCondition=0  SampleTime=2.26757369614512e-05
  PipelineRegister1 : Delay  DelayLength=double(1)  InitialCondition=0  SampleTime=2.26757369614512e-05
  Rate Transition : hdlmdlgenlib/Buffer
      settings: SourceProductBaseCode=SL
  delayMatch : Delay  DelayLength=double(1)  InitialCondition=0  SampleTime=2.26757369614512e-05
  Out_LoR_e : Outport  OutDataTypeStr=fixdt(0,16,25)  SampleTime=2.26757369614512e-05  VectorParamsAs1DForOutWhenUnconnected=off
  wires:
  Add/1 -> Out_LoR_e/1
  Constant10/1 -> HwModeRegister2/1
  Constant8/1 -> HwModeRegister/1
  Delay/1 -> Rate Transition/1
  PipelineRegister/1 -> Add/1
  delayMatch/1 -> Add/2
  Rate Transition/1 -> HwModeRegister3/1
  In_LoR_e/1 -> Delay/1, HwModeRegister1/1
  PipelineRegister1/1 -> delayMatch/1
  Multiply/1 -> PipelineRegister/1
  HwModeRegister/1 -> Multiply/1
  HwModeRegister1/1 -> Multiply/2
  Multiply1/1 -> PipelineRegister1/1
  HwModeRegister2/1 -> Multiply1/1
  HwModeRegister3/1 -> Multiply1/2

== system gm_final_heart_sym2_level4_hdl/DWT_Sym2_Level4/1st_Level_Recon/LoR_Odd ==
  In_LoR_o : Inport  OutDataTypeStr=fixdt(0, 16, 24)  PortDimensions=1  SampleTime=2.26757369614512e-05
  Add : Sum  AccumDataTypeStr=fixdt(1, 16, 23)  OutDataTypeStr=fixdt(1, 16, 24)  SampleTime=2.26757369614512e-05
  Constant11 : Constant  Value=-0.1294097900390625  OutDataTypeStr=fixdt(1, 16, 17)  SampleTime=2.26757369614512e-05
  Constant9 : Constant  Value=0.836517333984375  OutDataTypeStr=fixdt(0, 16, 16)  SampleTime=2.26757369614512e-05
  Delay : Delay  DelayLength=double(1)  InitialCondition=0  SampleTime=2.26757369614512e-05
  HwModeRegister{,1..3} (4 alike) : Delay  DelayLength=double(1)  InitialCondition=0  SampleTime=2.26757369614512e-05
  Multiply : Product  Inputs=**  OutDataTypeStr=fixdt(0, 16, 24)  SampleTime=2.26757369614512e-05
  Multiply1 : Product  Inputs=**  OutDataTypeStr=fixdt(1, 16, 15)  SampleTime=2.26757369614512e-05
  PipelineRegister : Delay  DelayLength=double(1)  InitialCondition=0  SampleTime=2.26757369614512e-05
  PipelineRegister1 : Delay  DelayLength=double(1)  InitialCondition=0  SampleTime=2.26757369614512e-05
  Rate Transition : hdlmdlgenlib/Buffer
      settings: SourceProductBaseCode=SL
  delayMatch : Delay  DelayLength=double(1)  InitialCondition=0  SampleTime=2.26757369614512e-05
  Out_HiR_o : Outport  OutDataTypeStr=fixdt(1,16,24)  SampleTime=2.26757369614512e-05  VectorParamsAs1DForOutWhenUnconnected=off
  wires:
  Add/1 -> Out_HiR_o/1
  Constant11/1 -> HwModeRegister2/1
  Constant9/1 -> HwModeRegister/1
  Delay/1 -> Rate Transition/1
  PipelineRegister/1 -> Add/1
  delayMatch/1 -> Add/2
  Rate Transition/1 -> HwModeRegister3/1
  In_LoR_o/1 -> Delay/1, HwModeRegister1/1
  PipelineRegister1/1 -> delayMatch/1
  Multiply/1 -> PipelineRegister/1
  HwModeRegister/1 -> Multiply/1
  HwModeRegister1/1 -> Multiply/2
  Multiply1/1 -> PipelineRegister1/1
  HwModeRegister2/1 -> Multiply1/1
  HwModeRegister3/1 -> Multiply1/2

== system gm_final_heart_sym2_level4_hdl/DWT_Sym2_Level4/1st_Level_Recon1/HiR_Even ==
  In_HiR_e : Inport  OutDataTypeStr=fixdt(1, 16, 27)  PortDimensions=1  SampleTime=2.26757369614512e-05
  Add : Sum  AccumDataTypeStr=fixdt(1, 16, 28)  OutDataTypeStr=fixdt(1, 16, 28)  SampleTime=2.26757369614512e-05
  Constant12 : Constant  Value=-0.1294097900390625  OutDataTypeStr=fixdt(1, 16, 17)  SampleTime=2.26757369614512e-05
  Constant14 : Constant  Value=0.836517333984375  OutDataTypeStr=fixdt(0, 16, 16)  SampleTime=2.26757369614512e-05
  Delay : Delay  DelayLength=double(1)  InitialCondition=0  SampleTime=2.26757369614512e-05
  HwModeRegister{,1..3} (4 alike) : Delay  DelayLength=double(1)  InitialCondition=0  SampleTime=2.26757369614512e-05
  Multiply : Product  Inputs=**  OutDataTypeStr=fixdt(1, 16, 30)  SampleTime=2.26757369614512e-05
  Multiply1 : Product  Inputs=**  OutDataTypeStr=fixdt(1, 16, 28)  SampleTime=2.26757369614512e-05
  PipelineRegister : Delay  DelayLength=double(1)  InitialCondition=0  SampleTime=2.26757369614512e-05
  PipelineRegister1 : Delay  DelayLength=double(1)  InitialCondition=0  SampleTime=2.26757369614512e-05
  Rate Transition : hdlmdlgenlib/Buffer
      settings: SourceProductBaseCode=SL
  delayMatch : Delay  DelayLength=double(1)  InitialCondition=0  SampleTime=2.26757369614512e-05
  Out_HiR_e : Outport  OutDataTypeStr=fixdt(1,16,28)  SampleTime=2.26757369614512e-05  VectorParamsAs1DForOutWhenUnconnected=off
  wires:
  Add/1 -> Out_HiR_e/1
  Constant12/1 -> HwModeRegister/1
  Constant14/1 -> HwModeRegister2/1
  Delay/1 -> Rate Transition/1
  PipelineRegister/1 -> Add/1
  delayMatch/1 -> Add/2
  Rate Transition/1 -> HwModeRegister3/1
  In_HiR_e/1 -> Delay/1, HwModeRegister1/1
  PipelineRegister1/1 -> delayMatch/1
  Multiply/1 -> PipelineRegister/1
  HwModeRegister/1 -> Multiply/1
  HwModeRegister1/1 -> Multiply/2
  Multiply1/1 -> PipelineRegister1/1
  HwModeRegister2/1 -> Multiply1/1
  HwModeRegister3/1 -> Multiply1/2

== system gm_final_heart_sym2_level4_hdl/DWT_Sym2_Level4/1st_Level_Recon1/HiR_Odd ==
  In_HiR_o : Inport  OutDataTypeStr=fixdt(1, 16, 27)  PortDimensions=1  SampleTime=2.26757369614512e-05
  Add : Sum  AccumDataTypeStr=fixdt(1, 16, 29)  OutDataTypeStr=fixdt(1, 16, 29)  SampleTime=2.26757369614512e-05
  Constant13 : Constant  Value=-0.22414398193359375  OutDataTypeStr=fixdt(1, 16, 17)  SampleTime=2.26757369614512e-05
  Constant15 : Constant  Value=-0.4829559326171875  OutDataTypeStr=fixdt(1, 16, 16)  SampleTime=2.26757369614512e-05
  Delay : Delay  DelayLength=double(1)  InitialCondition=0  SampleTime=2.26757369614512e-05
  HwModeRegister{,1..3} (4 alike) : Delay  DelayLength=double(1)  InitialCondition=0  SampleTime=2.26757369614512e-05
  Multiply : Product  Inputs=**  OutDataTypeStr=fixdt(1, 16, 30)  SampleTime=2.26757369614512e-05
  Multiply1 : Product  Inputs=**  OutDataTypeStr=fixdt(1, 16, 29)  SampleTime=2.26757369614512e-05
  PipelineRegister : Delay  DelayLength=double(1)  InitialCondition=0  SampleTime=2.26757369614512e-05
  PipelineRegister1 : Delay  DelayLength=double(1)  InitialCondition=0  SampleTime=2.26757369614512e-05
  Rate Transition : hdlmdlgenlib/Buffer
      settings: SourceProductBaseCode=SL
  delayMatch : Delay  DelayLength=double(1)  InitialCondition=0  SampleTime=2.26757369614512e-05
  Out_HiR_o : Outport  OutDataTypeStr=fixdt(1,16,29)  SampleTime=2.26757369614512e-05  VectorParamsAs1DForOutWhenUnconnected=off
  wires:
  Add/1 -> Out_HiR_o/1
  Constant13/1 -> HwModeRegister/1
  Constant15/1 -> HwModeRegister2/1
  Delay/1 -> Rate Transition/1
  PipelineRegister/1 -> Add/1
  delayMatch/1 -> Add/2
  Rate Transition/1 -> HwModeRegister3/1
  In_HiR_o/1 -> Delay/1, HwModeRegister1/1
  PipelineRegister1/1 -> delayMatch/1
  Multiply/1 -> PipelineRegister/1
  HwModeRegister/1 -> Multiply/1
  HwModeRegister1/1 -> Multiply/2
  Multiply1/1 -> PipelineRegister1/1
  HwModeRegister2/1 -> Multiply1/1
  HwModeRegister3/1 -> Multiply1/2

== system gm_final_heart_sym2_level4_hdl/DWT_Sym2_Level4/1st_Level_Recon1/LoR_Even ==
  In_LoR_e : Inport  OutDataTypeStr=fixdt(1, 16, 23)  PortDimensions=1  SampleTime=2.26757369614512e-05
  Add : Sum  AccumDataTypeStr=fixdt(1, 16, 23)  OutDataTypeStr=fixdt(1, 16, 23)  SampleTime=2.26757369614512e-05
  Constant10 : Constant  Value=0.22414398193359375  OutDataTypeStr=fixdt(0, 16, 18)  SampleTime=2.26757369614512e-05
  Constant8 : Constant  Value=0.48296356201171875  OutDataTypeStr=fixdt(0, 16, 17)  SampleTime=2.26757369614512e-05
  Delay : Delay  DelayLength=double(1)  InitialCondition=0  SampleTime=2.26757369614512e-05
  HwModeRegister{,1..3} (4 alike) : Delay  DelayLength=double(1)  InitialCondition=0  SampleTime=2.26757369614512e-05
  Multiply : Product  Inputs=**  OutDataTypeStr=fixdt(1, 16, 24)  SampleTime=2.26757369614512e-05
  Multiply1 : Product  Inputs=**  OutDataTypeStr=fixdt(1, 16, 25)  SampleTime=2.26757369614512e-05
  PipelineRegister : Delay  DelayLength=double(1)  InitialCondition=0  SampleTime=2.26757369614512e-05
  PipelineRegister1 : Delay  DelayLength=double(1)  InitialCondition=0  SampleTime=2.26757369614512e-05
  Rate Transition : hdlmdlgenlib/Buffer
      settings: SourceProductBaseCode=SL
  delayMatch : Delay  DelayLength=double(1)  InitialCondition=0  SampleTime=2.26757369614512e-05
  Out_LoR_e : Outport  OutDataTypeStr=fixdt(1,16,23)  SampleTime=2.26757369614512e-05  VectorParamsAs1DForOutWhenUnconnected=off
  wires:
  Add/1 -> Out_LoR_e/1
  Constant10/1 -> HwModeRegister2/1
  Constant8/1 -> HwModeRegister/1
  Delay/1 -> Rate Transition/1
  PipelineRegister/1 -> Add/1
  delayMatch/1 -> Add/2
  Rate Transition/1 -> HwModeRegister3/1
  In_LoR_e/1 -> Delay/1, HwModeRegister1/1
  PipelineRegister1/1 -> delayMatch/1
  Multiply/1 -> PipelineRegister/1
  HwModeRegister/1 -> Multiply/1
  HwModeRegister1/1 -> Multiply/2
  Multiply1/1 -> PipelineRegister1/1
  HwModeRegister2/1 -> Multiply1/1
  HwModeRegister3/1 -> Multiply1/2

== system gm_final_heart_sym2_level4_hdl/DWT_Sym2_Level4/1st_Level_Recon1/LoR_Odd ==
  In_LoR_o : Inport  OutDataTypeStr=fixdt(1, 16, 23)  PortDimensions=1  SampleTime=2.26757369614512e-05
  Add : Sum  AccumDataTypeStr=fixdt(1, 16, 23)  OutDataTypeStr=fixdt(1, 16, 23)  SampleTime=2.26757369614512e-05
  Constant11 : Constant  Value=-0.1294097900390625  OutDataTypeStr=fixdt(1, 16, 17)  SampleTime=2.26757369614512e-05
  Constant9 : Constant  Value=0.836517333984375  OutDataTypeStr=fixdt(0, 16, 16)  SampleTime=2.26757369614512e-05
  Delay : Delay  DelayLength=double(1)  InitialCondition=0  SampleTime=2.26757369614512e-05
  HwModeRegister{,1..3} (4 alike) : Delay  DelayLength=double(1)  InitialCondition=0  SampleTime=2.26757369614512e-05
  Multiply : Product  Inputs=**  OutDataTypeStr=fixdt(1, 16, 23)  SampleTime=2.26757369614512e-05
  Multiply1 : Product  Inputs=**  OutDataTypeStr=fixdt(1, 16, 26)  SampleTime=2.26757369614512e-05
  PipelineRegister : Delay  DelayLength=double(1)  InitialCondition=0  SampleTime=2.26757369614512e-05
  PipelineRegister1 : Delay  DelayLength=double(1)  InitialCondition=0  SampleTime=2.26757369614512e-05
  Rate Transition : hdlmdlgenlib/Buffer
      settings: SourceProductBaseCode=SL
  delayMatch : Delay  DelayLength=double(1)  InitialCondition=0  SampleTime=2.26757369614512e-05
  Out_HiR_o : Outport  OutDataTypeStr=fixdt(1,16,23)  SampleTime=2.26757369614512e-05  VectorParamsAs1DForOutWhenUnconnected=off
  wires:
  Add/1 -> Out_HiR_o/1
  Constant11/1 -> HwModeRegister2/1
  Constant9/1 -> HwModeRegister/1
  Delay/1 -> Rate Transition/1
  PipelineRegister/1 -> Add/1
  delayMatch/1 -> Add/2
  Rate Transition/1 -> HwModeRegister3/1
  In_LoR_o/1 -> Delay/1, HwModeRegister1/1
  PipelineRegister1/1 -> delayMatch/1
  Multiply/1 -> PipelineRegister/1
  HwModeRegister/1 -> Multiply/1
  HwModeRegister1/1 -> Multiply/2
  Multiply1/1 -> PipelineRegister1/1
  HwModeRegister2/1 -> Multiply1/1
  HwModeRegister3/1 -> Multiply1/2

== system gm_final_heart_sym2_level4_hdl/DWT_Sym2_Level4/1st_Level_Recon2/HiR_Even ==
  In_HiR_e : Inport  OutDataTypeStr=fixdt(1, 16, 27)  PortDimensions=1  SampleTime=2.26757369614512e-05
  Add : Sum  AccumDataTypeStr=fixdt(1, 16, 28)  OutDataTypeStr=fixdt(1, 16, 28)  SampleTime=2.26757369614512e-05
  Constant12 : Constant  Value=-0.1294097900390625  OutDataTypeStr=fixdt(1, 16, 17)  SampleTime=2.26757369614512e-05
  Constant14 : Constant  Value=0.836517333984375  OutDataTypeStr=fixdt(0, 16, 16)  SampleTime=2.26757369614512e-05
  Delay : Delay  DelayLength=double(1)  InitialCondition=0  SampleTime=2.26757369614512e-05
  HwModeRegister{,1..3} (4 alike) : Delay  DelayLength=double(1)  InitialCondition=0  SampleTime=2.26757369614512e-05
  Multiply : Product  Inputs=**  OutDataTypeStr=fixdt(1, 16, 30)  SampleTime=2.26757369614512e-05
  Multiply1 : Product  Inputs=**  OutDataTypeStr=fixdt(1, 16, 28)  SampleTime=2.26757369614512e-05
  PipelineRegister : Delay  DelayLength=double(1)  InitialCondition=0  SampleTime=2.26757369614512e-05
  PipelineRegister1 : Delay  DelayLength=double(1)  InitialCondition=0  SampleTime=2.26757369614512e-05
  Rate Transition : hdlmdlgenlib/Buffer
      settings: SourceProductBaseCode=SL
  delayMatch : Delay  DelayLength=double(1)  InitialCondition=0  SampleTime=2.26757369614512e-05
  Out_HiR_e : Outport  OutDataTypeStr=fixdt(1,16,28)  SampleTime=2.26757369614512e-05  VectorParamsAs1DForOutWhenUnconnected=off
  wires:
  Add/1 -> Out_HiR_e/1
  Constant12/1 -> HwModeRegister/1
  Constant14/1 -> HwModeRegister2/1
  Delay/1 -> Rate Transition/1
  PipelineRegister/1 -> Add/1
  delayMatch/1 -> Add/2
  Rate Transition/1 -> HwModeRegister3/1
  In_HiR_e/1 -> Delay/1, HwModeRegister1/1
  PipelineRegister1/1 -> delayMatch/1
  Multiply/1 -> PipelineRegister/1
  HwModeRegister/1 -> Multiply/1
  HwModeRegister1/1 -> Multiply/2
  Multiply1/1 -> PipelineRegister1/1
  HwModeRegister2/1 -> Multiply1/1
  HwModeRegister3/1 -> Multiply1/2

== system gm_final_heart_sym2_level4_hdl/DWT_Sym2_Level4/1st_Level_Recon2/HiR_Odd ==
  In_HiR_o : Inport  OutDataTypeStr=fixdt(1, 16, 27)  PortDimensions=1  SampleTime=2.26757369614512e-05
  Add : Sum  AccumDataTypeStr=fixdt(1, 16, 29)  OutDataTypeStr=fixdt(1, 16, 29)  SampleTime=2.26757369614512e-05
  Constant13 : Constant  Value=-0.22414398193359375  OutDataTypeStr=fixdt(1, 16, 17)  SampleTime=2.26757369614512e-05
  Constant15 : Constant  Value=-0.4829559326171875  OutDataTypeStr=fixdt(1, 16, 16)  SampleTime=2.26757369614512e-05
  Delay : Delay  DelayLength=double(1)  InitialCondition=0  SampleTime=2.26757369614512e-05
  HwModeRegister{,1..3} (4 alike) : Delay  DelayLength=double(1)  InitialCondition=0  SampleTime=2.26757369614512e-05
  Multiply : Product  Inputs=**  OutDataTypeStr=fixdt(1, 16, 30)  SampleTime=2.26757369614512e-05
  Multiply1 : Product  Inputs=**  OutDataTypeStr=fixdt(1, 16, 29)  SampleTime=2.26757369614512e-05
  PipelineRegister : Delay  DelayLength=double(1)  InitialCondition=0  SampleTime=2.26757369614512e-05
  PipelineRegister1 : Delay  DelayLength=double(1)  InitialCondition=0  SampleTime=2.26757369614512e-05
  Rate Transition : hdlmdlgenlib/Buffer
      settings: SourceProductBaseCode=SL
  delayMatch : Delay  DelayLength=double(1)  InitialCondition=0  SampleTime=2.26757369614512e-05
  Out_HiR_o : Outport  OutDataTypeStr=fixdt(1,16,29)  SampleTime=2.26757369614512e-05  VectorParamsAs1DForOutWhenUnconnected=off
  wires:
  Add/1 -> Out_HiR_o/1
  Constant13/1 -> HwModeRegister/1
  Constant15/1 -> HwModeRegister2/1
  Delay/1 -> Rate Transition/1
  PipelineRegister/1 -> Add/1
  delayMatch/1 -> Add/2
  Rate Transition/1 -> HwModeRegister3/1
  In_HiR_o/1 -> Delay/1, HwModeRegister1/1
  PipelineRegister1/1 -> delayMatch/1
  Multiply/1 -> PipelineRegister/1
  HwModeRegister/1 -> Multiply/1
  HwModeRegister1/1 -> Multiply/2
  Multiply1/1 -> PipelineRegister1/1
  HwModeRegister2/1 -> Multiply1/1
  HwModeRegister3/1 -> Multiply1/2

== system gm_final_heart_sym2_level4_hdl/DWT_Sym2_Level4/1st_Level_Recon2/LoR_Even ==
  In_LoR_e : Inport  OutDataTypeStr=fixdt(1, 16, 23)  PortDimensions=1  SampleTime=2.26757369614512e-05
  Add : Sum  AccumDataTypeStr=fixdt(1, 16, 23)  OutDataTypeStr=fixdt(1, 16, 23)  SampleTime=2.26757369614512e-05
  Constant10 : Constant  Value=0.22414398193359375  OutDataTypeStr=fixdt(0, 16, 18)  SampleTime=2.26757369614512e-05
  Constant8 : Constant  Value=0.48296356201171875  OutDataTypeStr=fixdt(0, 16, 17)  SampleTime=2.26757369614512e-05
  Delay : Delay  DelayLength=double(1)  InitialCondition=0  SampleTime=2.26757369614512e-05
  HwModeRegister{,1..3} (4 alike) : Delay  DelayLength=double(1)  InitialCondition=0  SampleTime=2.26757369614512e-05
  Multiply : Product  Inputs=**  OutDataTypeStr=fixdt(1, 16, 24)  SampleTime=2.26757369614512e-05
  Multiply1 : Product  Inputs=**  OutDataTypeStr=fixdt(1, 16, 25)  SampleTime=2.26757369614512e-05
  PipelineRegister : Delay  DelayLength=double(1)  InitialCondition=0  SampleTime=2.26757369614512e-05
  PipelineRegister1 : Delay  DelayLength=double(1)  InitialCondition=0  SampleTime=2.26757369614512e-05
  Rate Transition : hdlmdlgenlib/Buffer
      settings: SourceProductBaseCode=SL
  delayMatch : Delay  DelayLength=double(1)  InitialCondition=0  SampleTime=2.26757369614512e-05
  Out_LoR_e : Outport  OutDataTypeStr=fixdt(1,16,23)  SampleTime=2.26757369614512e-05  VectorParamsAs1DForOutWhenUnconnected=off
  wires:
  Add/1 -> Out_LoR_e/1
  Constant10/1 -> HwModeRegister2/1
  Constant8/1 -> HwModeRegister/1
  Delay/1 -> Rate Transition/1
  PipelineRegister/1 -> Add/1
  delayMatch/1 -> Add/2
  Rate Transition/1 -> HwModeRegister3/1
  In_LoR_e/1 -> Delay/1, HwModeRegister1/1
  PipelineRegister1/1 -> delayMatch/1
  Multiply/1 -> PipelineRegister/1
  HwModeRegister/1 -> Multiply/1
  HwModeRegister1/1 -> Multiply/2
  Multiply1/1 -> PipelineRegister1/1
  HwModeRegister2/1 -> Multiply1/1
  HwModeRegister3/1 -> Multiply1/2
